simulink model "STEP1_W"  (Simulink 8.4)
settings: Solver=ode45  SolverMode=SingleTasking  StartTime=0.0  StopTime=inf  FixedStep=2/64e5  RelTol=1e-3
values from neighbouring files (symbols this model uses):
  c = (U_E025^2-U_ES^2)/U_NG025^2    [Digital_AM_SNR_to_BER.m]    (also in KOSZI_P.m = menu('Kanalwahl','1-Kanal','2-Kanal','3-Kanal'); exercise_00.m = 300000000)
libraries: measurement_tools x3, dsparch4 x2, dspvision x2, system_blocks x1, dspsigops x1, dspsnks4 x1
settings Model: Creator=Schoenen  LastModifiedBy=Schoenen
settings DataIOCC: SignalLoggingName=sigsOut
settings OptimizationCC: ExpressionDepthLimit=128
settings DebuggingCC: SaveWithParameterizedLinksMsg=none  SignalResolutionControl=TryResolveAllWithWarning  SolverPrmCheckMsg=none  MultiTaskDSMMsg=warning  MultiTaskCondExecSysMsg=none  FcnCallInpInsideContextMsg=EnableAllAsError  StateNameClashWarn=none
settings HardwareCC: TargetUnknown=on
settings RTWCC: IncludeERTFirstTime=on

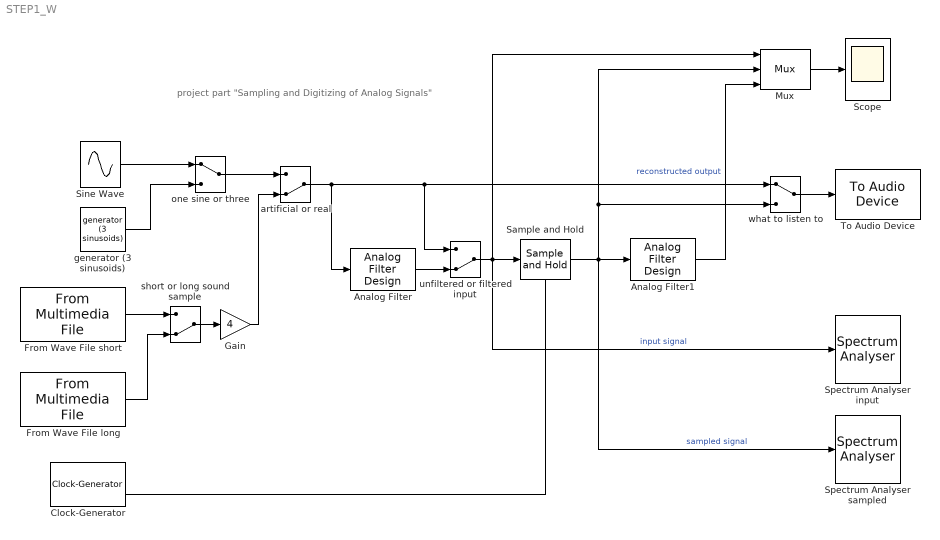
== system STEP1_W ==
  note: project part "Sampling and Digitizing of Analog Signals"
  Analog Filter : dsparch4/Analog Filter Design  method=Butterworth  filttype=Lowpass  N=24  Wlo=2*pi*c.filter_cutoff_frequency  Whi=80  Rp=2  Rs=40
  Analog Filter1 : dsparch4/Analog Filter Design  method=Butterworth  filttype=Lowpass  N=24  Wlo=2*pi*c.filter_cutoff_frequency  Whi=80  Rp=2  Rs=40
  Clock-Generator : system_blocks/Clock-Generator  bt=c.bit_clock_frequency  sr=c.sampling_frequency
  From Wave File long : dspvision/From Multimedia File  inputFilename=audio_sampled_with_8kHz.wav  loop=on  numPlays=1  outputStreams=Audio only  videoDataType=single  audioDataType=double  inheritSampleTime=on  userDefinedSampleTime=1/30  noAudioOutput=off  isIntensityVideo=off  fourcc=RGB  colorVideoFormat=Separate color signals  outputEOF=off  dataOrg=Column-major  audioFrameSize=1  computeAudioFrameSize=off  outSamplingMode=Sample based
  From Wave File short : dspvision/From Multimedia File  inputFilename=audio_in_8kHz.wav  loop=on  numPlays=1  outputStreams=Audio only  videoDataType=single  audioDataType=double  inheritSampleTime=on  userDefinedSampleTime=1/30  noAudioOutput=off  isIntensityVideo=off  fourcc=RGB  colorVideoFormat=Separate color signals  outputEOF=off  dataOrg=Column-major  audioFrameSize=1  computeAudioFrameSize=off  outSamplingMode=Sample based
  Gain : Gain  Gain=4
  Mux : Mux  Inputs=3
  Sample and Hold : dspsigops/Sample and Hold  trig=Rising edge  initCond=0  latchinput=off
  Scope : Scope
      settings: TimeRange=1  YMin=-1  YMax=1
  Sine Wave : Sin  Frequency=2*pi*1000  SampleTime=0
  Spectrum Analyser input : measurement_tools/Spectrum Analyser  st=c.sample_time
  Spectrum Analyser sampled : measurement_tools/Spectrum Analyser  st=c.sample_time/4
  To Audio Device : dspsnks4/To Audio Device  deviceName=Default  inheritSampleRate=off  sampleRate=8000  deviceDatatype=Determine from input data type  autoBufferSize=on  bufferSize=4096  queueDuration=1.0  defaultOutputChannelMapping=on  outputChannelMapping=1:2  outputNumUnderrunSamples=off
  artificial or real : ManualSwitch  CurrentSetting=0
  generator (3 sinusoids) : measurement_tools/generator (3 sinusoids)  MaskParam1="[1  1000  0]"  MaskParam2="[0.5  2000  0]"  MaskParam3="[0.25  3000  0]"
  one sine or three : ManualSwitch
  short or long sound sample : ManualSwitch  CurrentSetting=0
  unfiltered or filtered input : ManualSwitch  CurrentSetting=0
  what to listen to : ManualSwitch
  wires:
  Sine Wave/1 -> one sine or three/1
  generator (3 sinusoids)/1 -> one sine or three/2
  one sine or three/1 -> artificial or real/1
  From Wave File short/1 -> short or long sound sample/1
  From Wave File long/1 -> short or long sound sample/2
  artificial or real/1 -> what to listen to/1, unfiltered or filtered input/1, Analog Filter/1
  what to listen to/1 -> To Audio Device/1
  Analog Filter/1 -> unfiltered or filtered input/2
  unfiltered or filtered input/1 -> Spectrum Analyser input/1, Mux/1, Sample and Hold/1  "input signal"
  Clock-Generator/2 -> Sample and Hold/Trigger
  Mux/1 -> Scope/1
  Sample and Hold/1 -> Spectrum Analyser sampled/1, Analog Filter1/1, what to listen to/2, Mux/2  "sampled signal"
  Analog Filter1/1 -> Mux/3  "reconstructed output"
  short or long sound sample/1 -> Gain/1
  Gain/1 -> artificial or real/2
